simulink model "GalvoModel_simo_ss"  (R2013a)
settings: Solver=ode45  StartTime=0.0  StopTime=10.0  RelTol=1e-3
values from neighbouring files (symbols this model uses):
  Lc = 170e-6    (= 0.00017)    [Galvo_process_analyze.m]
  Rc = 1.5    [Galvo_process_analyze.m]
undefined symbols (not defined in the file or in its folder): JR, KBM, KFR, KMT, KTB, Rsh
settings Model: Creator=mainster  LastModifiedBy=mainster

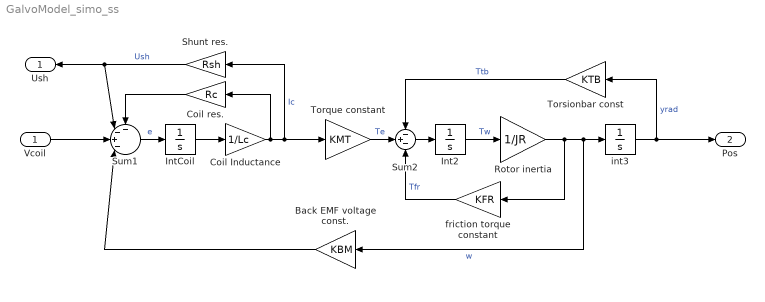
== system GalvoModel_simo_ss ==
  Vcoil : Inport
  Back EMF voltage const. : Gain  Gain=KBM
  Coil Inductance : Gain  Gain=1/Lc
  Coil res. : Gain  Gain=Rc
  Int2 : Integrator
  IntCoil : Integrator
  Rotor inertia : Gain  Gain=1/JR
  Shunt res. : Gain  Gain=Rsh
  Sum1 : Sum  Inputs=--+-|
  Sum2 : Sum  Inputs=-+-
  Torque constant : Gain  Gain=KMT
  Torsionbar const : Gain  Gain=KTB
  friction torque constant : Gain  Gain=KFR
  int3 : Integrator
  Ush : Outport
  Pos : Outport  Port=2
  wires:
  Shunt res./1 -> Ush/1, Sum1/2  "Ush"
  Coil res./1 -> Sum1/1
  Vcoil/1 -> Sum1/3
  Back EMF voltage const./1 -> Sum1/4
  int3/1 -> Pos/1, Torsionbar const/1  "yrad"
  Torque constant/1 -> Sum2/2  "Te"
  Coil Inductance/1 -> Shunt res./1, Torque constant/1, Coil res./1  "Ic"
  Torsionbar const/1 -> Sum2/1  "Ttb"
  IntCoil/1 -> Coil Inductance/1
  Sum1/1 -> IntCoil/1  "e"
  Int2/1 -> Rotor inertia/1  "Tw"
  Sum2/1 -> Int2/1
  Rotor inertia/1 -> int3/1, Back EMF voltage const./1, friction torque constant/1  "w"
  friction torque constant/1 -> Sum2/3  "Tfr"
